simulink model "PID_DC_MotorControl_Enc"  (R2021b)
settings: Solver=FixedStepAuto  StartTime=0.0  StopTime=inf  RelTol=1e-3  EnableMultiTasking=on
libraries: arduinolib x3, arduinosensorlib x1, simulink x1
settings Model: ExtModeTrigDuration=2  Creator=Ghani  LastModifiedBy=Ghani
settings SolverCC: AutoInsertRateTranBlk=on
settings OptimizationCC: EnhancedBackFolding=on  PassReuseOutputArgsAs=Individual arguments  ZeroExternalMemoryAtStartup=off  ZeroInternalMemoryAtStartup=off  MaxStackSize=64  OptimizeBlockOrder=speed  DifferentSizesBufferReuse=on  OptimizationCustomize=off  EfficientTunableParamExpr=on
settings DebuggingCC: ParameterTunabilityLossMsg=error
settings HardwareCC: ProdBitPerPointer=32  ProdBitPerSizeT=32  ProdBitPerPtrDiffT=32  ProdLargestAtomicInteger=Long  ProdLargestAtomicFloat=Double  ProdWordSize=32  ProdHWDeviceType=ARM Compatible->ARM Cortex  UseEmbeddedCoderFeatures=off  UseSimulinkCoderFeatures=off
settings SFSimCC: MATLABDynamicMemAlloc=off
settings RTWCC: Description=Embedded Coder  SystemTargetFile=ert.tlc  HardwareBoard=Arduino Due  TemplateMakefile=ert_default_tmf  Toolchain=Arduino ARM  BuildConfiguration=Faster Runs
settings CodeAppCC: ForceParamTrailComments=on  IgnoreCustomStorageClasses=off  OperatorAnnotations=on  SimulinkDataObjDesc=on  SFDataObjDesc=on  InsertBlockDesc=on
settings ERTTargetCC: SupportContinuousTime=on  SupportNonInlinedSFcns=on  SupportVariableSizeSignals=on  ExtModeTransport=3  ExtModeStaticAlloc=on  ExtModeStaticAllocSize=24576  ExtModeMexFile=ext_xcp  ExtModeIntrfLevel=Level2 - Open

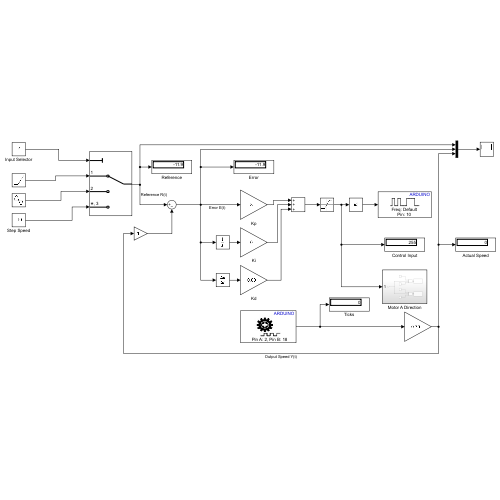
[thumbnail: Simulink's stored preview of the top-level diagram]
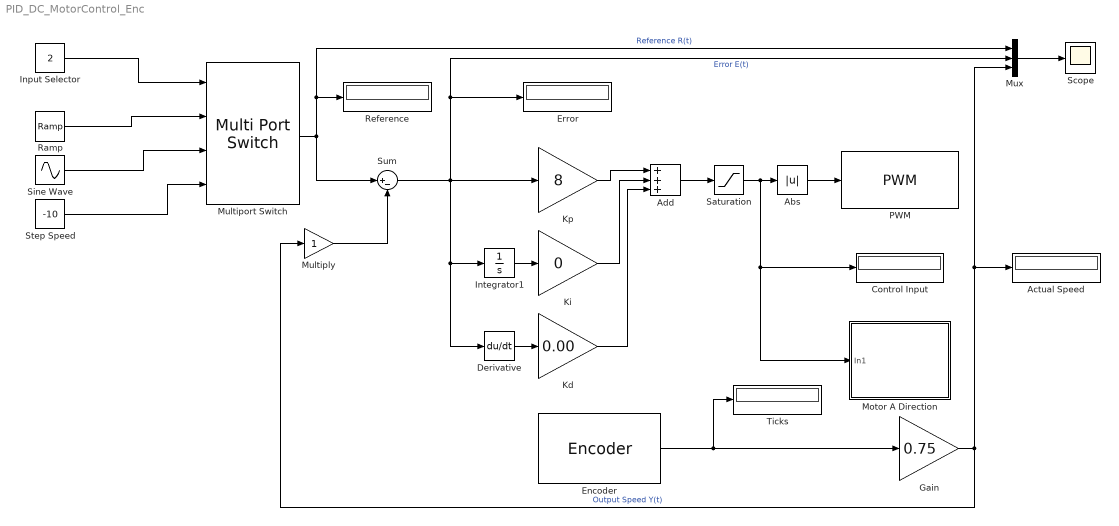
== system PID_DC_MotorControl_Enc ==
  Abs : Abs
  Actual Speed : Display
  Add : Sum  Inputs=+++
  Control Input : Display
  Derivative : Derivative
  Encoder : arduinosensorlib/Encoder  InputA=2  InputB=18  Mode=Reset at each Sample time  SampleTime=0.02
      settings: SourceProductBaseCode=ARDUINO
  Error : Display
  Gain : Gain  Gain=0.75  OutDataTypeStr=double  RndMeth=Nearest
  Input Selector : Constant  Value=2
  Integrator1 : Integrator
  Kd : Gain  Gain=0.00
  Ki : Gain  Gain=0
  Kp : Gain  Gain=8
  Motor A Direction : Subsystem
  Multiply : Gain
  Multiport Switch : MultiPortSwitch
  Mux : Mux  Inputs=3
  PWM : arduinolib/PWM  pinNumber=10  frequencyType=Default  desiredFrequency=490.2  achievableFrequency=490.2
  Ramp : simulink/Sources/Ramp  slope=1  start=0  InitialOutput=0
  Reference : Display
  Saturation : Saturate  UpperLimit=255  LowerLimit=-255
  Scope : Scope
  Sine Wave : Sin  Amplitude=100  SampleTime=0
  Step Speed : Constant  Value=-10
  Sum : Sum  Inputs=|+-
  Ticks : Display
  wires:
  Kp/1 -> Add/1
  Encoder/1 -> Ticks/1, Gain/1
  Gain/1 -> Multiply/1, Mux/3, Actual Speed/1  "Output Speed Y(t)"
  Sum/1 -> Error/1, Mux/2, Kp/1, Derivative/1, Integrator1/1  "Error E(t)"
  Mux/1 -> Scope/1
  Integrator1/1 -> Ki/1
  Ki/1 -> Add/2
  Add/1 -> Saturation/1
  Saturation/1 -> Control Input/1, Motor A Direction/1(In1), Abs/1
  Abs/1 -> PWM/1
  Multiply/1 -> Sum/2
  Sine Wave/1 -> Multiport Switch/3
  Step Speed/1 -> Multiport Switch/4
  Multiport Switch/1 -> Mux/1, Reference/1, Sum/1  "Reference R(t)"
  Derivative/1 -> Kd/1
  Kd/1 -> Add/3
  Ramp/1 -> Multiport Switch/2
  Input Selector/1 -> Multiport Switch/1

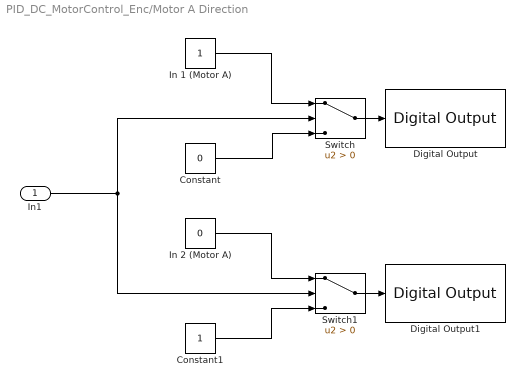
== system PID_DC_MotorControl_Enc/Motor A Direction ==
  In1 : Inport
  Constant : Constant  Value=0
  Constant1 : Constant
  Digital Output : arduinolib/Digital Output  pinNumber=4  Direction=output  blockPlatform=arduino
  Digital Output1 : arduinolib/Digital Output  pinNumber=5  Direction=output  blockPlatform=arduino
  In 1 (Motor A) : Constant
  In 2 (Motor A) : Constant  Value=0
  Switch : Switch  Criteria=u2 > Threshold
  Switch1 : Switch  Criteria=u2 > Threshold
  wires:
  In 2 (Motor A)/1 -> Switch1/1
  In 1 (Motor A)/1 -> Switch/1
  Switch/1 -> Digital Output/1
  Switch1/1 -> Digital Output1/1
  Constant/1 -> Switch/3
  Constant1/1 -> Switch1/3
  In1/1 -> Switch1/2, Switch/2
